simulink library "libtb_gen_canMsgCntr"  (R2020a)
settings: Solver=VariableStepAuto  StartTime=0.0  StopTime=10.0  RelTol=1e-3  EnableMultiTasking=on
settings Model: Creator=home  LastModifiedBy=Administrator
settings DataIOCC: LimitDataPoints=on  ReturnWorkspaceOutputs=off
settings OptimizationCC: LifeSpan=inf
settings DebuggingCC: AllowSymbolicDim=off  SFUnexpectedBacktrackingDiag=warning  SFNoUnconditionalDefaultTransitionDiag=warning  SFExecutionAtInitializationDiag=none  ArithmeticOperatorsInVariantConditions=warning
settings ModelReferenceCC: PropagateSignalLabelsOutOfModel=off
settings SFSimCC: SimUseLocalCustomCode=off  CustomCodeUndefinedFunction=UseInterfaceOnly
settings RTWCC: RTWUseLocalCustomCode=off
settings CodeAppCC: StateflowObjectComments=on
settings GRTTargetCC: TargetLangStandard=C89/C90 (ANSI)
settings ConfigComp: CovMetricSettings=dw  CovHtmlReporting=on  CovSaveCumulativeToWorkspaceVar=on  CovSaveSingleToWorkspaceVar=on  CovExternalEMLEnable=off

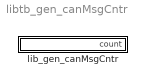
== system libtb_gen_canMsgCntr ==
  lib_gen_canMsgCntr : Stateflow chart  TreatAsAtomicUnit=on

== stateflow chart libtb_gen_canMsgCntr/lib_gen_canMsgCntr ==
  state counter
  (default) -> counter : { count = 0}
  counter -> (junction 5) : {count = count+1;}
  (junction 5) -> counter [order 2]
  (junction 5) -> counter [order 1] : [count > 15] {count = 0;}
  data: count output uint8
  events: event input RISING_EDGE_EVENT
